simulink model "simuDosValvula"  (R2018a)
settings: Solver=VariableStepAuto  StartTime=0.0  StopTime=2  RelTol=1e-3
libraries: simulink x2, pePwmGenerator x2, vrlib x1
settings Model: Creator=Ruben  LastModifiedBy=Ruben

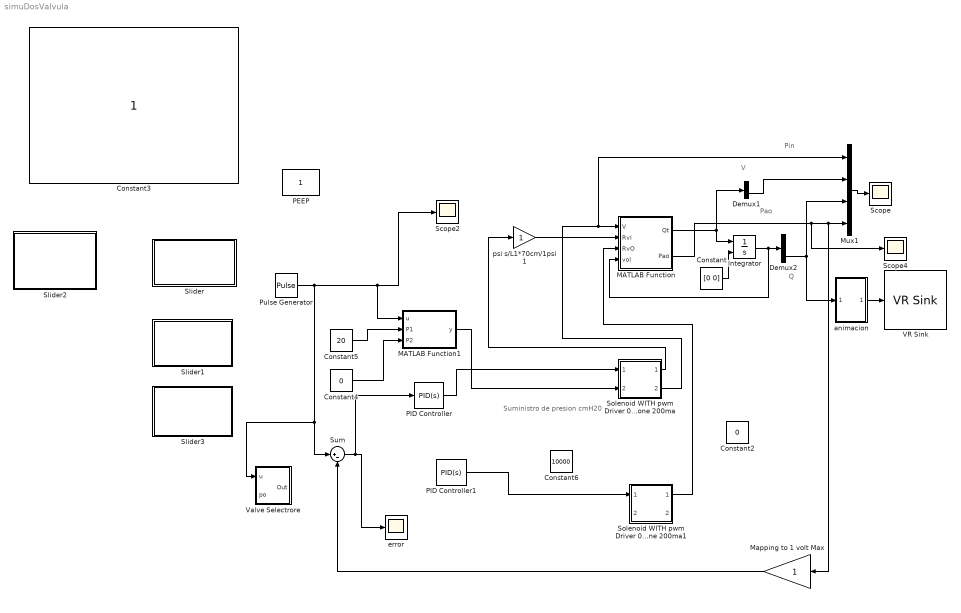
== system simuDosValvula ==
  note: Suministro de presion
      | cmH20
  note: Q
  note: Pin
  note: V
  note: Pao
  Constant : Constant  Value="[0    0]"
  Constant2 : Constant  Value=0
  Constant3 : Constant
      mask Display: image('C:\Users\Ruben\Downloads\Equivalente.png');
  Constant4 : Constant  Value=0
  Constant5 : Constant  Value=20
  Constant6 : Constant  Value=10000
  Demux1 : Demux  Outputs=2
  Demux2 : Demux  Outputs=2
  Integrator : Integrator  InitialConditionSource=external
  MATLAB Function : MATLAB Function  TreatAsAtomicUnit=on
  MATLAB Function1 : MATLAB Function  TreatAsAtomicUnit=on
  Mapping to 1 volt Max : Gain
  Mux1 : Mux
  PEEP : Constant
  PID Controller : simulink/Continuous/PID Controller  Controller=PID  TimeDomain=Continuous-time  SampleTime=-1  IntegratorMethod=Forward Euler  FilterMethod=Forward Euler  Form=Parallel  UseFilter=on  ControllerParametersSource=internal  P=.05  I=0  D=0  N=100  InitialConditionSource=internal  InitialConditionForIntegrator=0  InitialConditionForFilter=0  ExternalReset=none  LimitOutput=on  UpperSaturationLimit=1  LowerSaturationLimit=0  LinearizeAsGain=on  AntiWindupMode=none  Kb=1  TrackingMode=off  Kt=1  PParamMin=[]  PParamMax=[]  IParamMin=[]  IParamMax=[]  DParamMin=[]  DParamMax=[]  NParamMin=[]  NParamMax=[]  KbParamMin=[]  KbParamMax=[]  KtParamMin=[]  KtParamMax=[]  POutMin=[]  POutMax=[]  IOutMin=[]  IOutMax=[]  DOutMin=[]  DOutMax=[]  NOutMin=[]  NOutMax=[]  KbOutMin=[]  KbOutMax=[]  KtOutMin=[]  KtOutMax=[]  IntegratorOutMin=[]  IntegratorOutMax=[]  FilterOutMin=[]  FilterOutMax=[]  SumOutMin=[]  SumOutMax=[]  SumI1OutMin=[]  SumI1OutMax=[]  SumI2OutMin=[]  SumI2OutMax=[]  SumI3OutMin=[]  SumI3OutMax=[]  SumDOutMin=[]  SumDOutMax=[]  SaturationOutMin=[]  SaturationOutMax=[]  IntegratorContinuousStateAttributes=''  IntegratorStateMustResolveToSignalObject=off  IntegratorRTWStateStorageClass=Auto  FilterContinuousStateAttributes=''  FilterStateMustResolveToSignalObject=off  FilterRTWStateStorageClass=Auto  DifferentiatorICPrevScaledInput=0  DifferentiatorOutMin=[]  DifferentiatorOutMax=[]  FilterDiffOutCoefMin=[]  FilterDiffOutCoefMax=[]  SumDenOutMin=[]  SumDenOutMax=[]  SumNumOutMin=[]  SumNumOutMax=[]  ReciprocalOutMin=[]  ReciprocalOutMax=[]  DivideOutMin=[]  DivideOutMax=[]  TunerSelectOption=Transfer Function Based (PID Tuner App)
  PID Controller1 : simulink/Continuous/PID Controller  Controller=PID  TimeDomain=Continuous-time  SampleTime=-1  IntegratorMethod=Forward Euler  FilterMethod=Forward Euler  Form=Parallel  UseFilter=on  ControllerParametersSource=internal  P=1  I=0  D=0  N=100  InitialConditionSource=internal  InitialConditionForIntegrator=0  InitialConditionForFilter=0  ExternalReset=none  LimitOutput=on  UpperSaturationLimit=1  LowerSaturationLimit=0  LinearizeAsGain=on  AntiWindupMode=none  Kb=1  TrackingMode=off  Kt=1  PParamMin=[]  PParamMax=[]  IParamMin=[]  IParamMax=[]  DParamMin=[]  DParamMax=[]  NParamMin=[]  NParamMax=[]  KbParamMin=[]  KbParamMax=[]  KtParamMin=[]  KtParamMax=[]  POutMin=[]  POutMax=[]  IOutMin=[]  IOutMax=[]  DOutMin=[]  DOutMax=[]  NOutMin=[]  NOutMax=[]  KbOutMin=[]  KbOutMax=[]  KtOutMin=[]  KtOutMax=[]  IntegratorOutMin=[]  IntegratorOutMax=[]  FilterOutMin=[]  FilterOutMax=[]  SumOutMin=[]  SumOutMax=[]  SumI1OutMin=[]  SumI1OutMax=[]  SumI2OutMin=[]  SumI2OutMax=[]  SumI3OutMin=[]  SumI3OutMax=[]  SumDOutMin=[]  SumDOutMax=[]  SaturationOutMin=[]  SaturationOutMax=[]  IntegratorContinuousStateAttributes=''  IntegratorStateMustResolveToSignalObject=off  IntegratorRTWStateStorageClass=Auto  FilterContinuousStateAttributes=''  FilterStateMustResolveToSignalObject=off  FilterRTWStateStorageClass=Auto  DifferentiatorICPrevScaledInput=0  DifferentiatorOutMin=[]  DifferentiatorOutMax=[]  FilterDiffOutCoefMin=[]  FilterDiffOutCoefMax=[]  SumDenOutMin=[]  SumDenOutMax=[]  SumNumOutMin=[]  SumNumOutMax=[]  ReciprocalOutMin=[]  ReciprocalOutMax=[]  DivideOutMin=[]  DivideOutMax=[]  TunerSelectOption=Transfer Function Based (PID Tuner App)
  Pulse Generator : DiscretePulseGenerator  PulseType=Time based  Amplitude=10  Period=4  PulseWidth=30
  Scope : Scope
  Scope2 : Scope
  Scope4 : Scope
  Slider : Subsystem  DialogController=hmiCreateDDGDialog  IsWebBlock=on  mask(MWDashboardBlock){webBlockId=5c75009d-8c8d-43fb-88f0-46defad8d923, webBlockType=slider, ShowInLibBrowser=on, ShowInitialText=on, HMISrcModelName=simuDosValvula}
      mask prompts: webBlockId "WebBlock Id"; webBlockType "WebBlock Type"; HMISrcModelName "Source Model"
      mask help: SimulinkHMI:dialogs:SliderDialogDesc
      mask Help: helpview([docroot '/mapfiles/simulink.map'], 'hmi_slider')
      mask Display:
      | if strcmp(get_param(bdroot(gcb),'BlockDiagramType'), 'library')
      |     image([(matlabroot) '/toolbox/simulink/hmi/icons/Slider.png']);
      | end
  Slider1 : Subsystem  DialogController=hmiCreateDDGDialog  IsWebBlock=on  mask(MWDashboardBlock){webBlockId=99f10f40-54f3-4e18-818e-e2eb05ba8e4b, webBlockType=slider, ShowInLibBrowser=on, ShowInitialText=on, HMISrcModelName=simuDosValvula}
      mask prompts: webBlockId "WebBlock Id"; webBlockType "WebBlock Type"; HMISrcModelName "Source Model"
      mask help: SimulinkHMI:dialogs:SliderDialogDesc
      mask Help: helpview([docroot '/mapfiles/simulink.map'], 'hmi_slider')
      mask Display:
      | if strcmp(get_param(bdroot(gcb),'BlockDiagramType'), 'library')
      |     image([(matlabroot) '/toolbox/simulink/hmi/icons/Slider.png']);
      | end
  Slider2 : Subsystem  DialogController=hmiCreateDDGDialog  IsWebBlock=on  mask(MWDashboardBlock){webBlockId=e22ecaa3-1780-4869-841e-5d5c93829daa, webBlockType=slider, ShowInLibBrowser=on, ShowInitialText=on, HMISrcModelName=simuDosValvula}
      mask prompts: webBlockId "WebBlock Id"; webBlockType "WebBlock Type"; HMISrcModelName "Source Model"
      mask help: SimulinkHMI:dialogs:SliderDialogDesc
      mask Help: helpview([docroot '/mapfiles/simulink.map'], 'hmi_slider')
      mask Display:
      | if strcmp(get_param(bdroot(gcb),'BlockDiagramType'), 'library')
      |     image([(matlabroot) '/toolbox/simulink/hmi/icons/Slider.png']);
      | end
  Slider3 : Subsystem  DialogController=hmiCreateDDGDialog  IsWebBlock=on  mask(MWDashboardBlock){webBlockId=ff860e86-57b2-4262-afc4-ebabe2220a1a, webBlockType=slider, ShowInLibBrowser=on, ShowInitialText=on, HMISrcModelName=simuDosValvula}
      mask prompts: webBlockId "WebBlock Id"; webBlockType "WebBlock Type"; HMISrcModelName "Source Model"
      mask help: SimulinkHMI:dialogs:SliderDialogDesc
      mask Help: helpview([docroot '/mapfiles/simulink.map'], 'hmi_slider')
      mask Display:
      | if strcmp(get_param(bdroot(gcb),'BlockDiagramType'), 'library')
      |     image([(matlabroot) '/toolbox/simulink/hmi/icons/Slider.png']);
      | end
  Solenoid WITH pwm Driver 0v  closed to 1v fully  open min Resi=0.366 at 600ma (1 volt) dead zone 200ma : Subsystem  TreatAsAtomicUnit=on
      mask Display: image('C:\Users\Ruben\Downloads\Proportional-Safety_Valve.jpg');
  Solenoid WITH pwm Driver 0v  closed to 1v fully  open min Resi=0.366 at 600ma (1 volt) dead zone 200ma1 : Subsystem  TreatAsAtomicUnit=on
      mask Display: image('C:\Users\Ruben\Downloads\Proportional-Safety_Valve.jpg');
  Sum : Sum  Inputs=|+-
  VR Sink : vrlib/VR Sink  InstantiateOnLoad=on  SampleTime=0.1  ViewEnable=on  RemoteChange=off  RemoteView=off  FieldsWritten=lungs.scale.3.1.1.double  WorldFileName=Lungs2.wrl  AutoView=off  VideoDimensions=[]  AllowVariableSize=off  mask(Virtual Reality Sink){}
      settings: SourceProductBaseCode=VR
      mask Display: image('C:\Users\Ruben\Downloads\animacion.png');
  Valve Selectrore : MATLAB Function  TreatAsAtomicUnit=on
  animacion : Subsystem  TreatAsAtomicUnit=on
  error : Scope
  psi s/L1*70cm/1psi 1 : Gain
  wires:
  MATLAB Function/1(Qt) -> Integrator/1, Demux1/1
  Integrator/1 -> Demux2/1, MATLAB Function/4(vol)
  Constant/1 -> Integrator/2
  Solenoid WITH pwm Driver 0v  closed to 1v fully  open min Resi=0.366 at 600ma (1 volt) dead zone 200ma/1(Req(PSI.min/L)ma) -> psi s/L1*70cm/1psi 1/1
  psi s/L1*70cm/1psi 1/1 -> MATLAB Function/2(RvI)
  MATLAB Function1/1(y) -> Solenoid WITH pwm Driver 0v  closed to 1v fully  open min Resi=0.366 at 600ma (1 volt) dead zone 200ma/2(Pesion)
  Demux2/2 -> animacion/1(In1), Mux1/3
  Mux1/1 -> Scope/1
  Demux1/2 -> Mux1/2
  animacion/1(Out1) -> VR Sink/1
  Solenoid WITH pwm Driver 0v  closed to 1v fully  open min Resi=0.366 at 600ma (1 volt) dead zone 200ma/2(Presion) -> Mux1/1, MATLAB Function/1(V)
  Pulse Generator/1 -> Valve Selectrore/1(u), Sum/1, MATLAB Function1/1(u), Scope2/1
  MATLAB Function/2(Pao) -> Scope4/1, Mapping to 1 volt Max/1, Mux1/4
  Constant4/1 -> MATLAB Function1/3(P2)
  Constant5/1 -> MATLAB Function1/2(P1)
  Mapping to 1 volt Max/1 -> Sum/2
  Sum/1 -> PID Controller/1, error/1
  Solenoid WITH pwm Driver 0v  closed to 1v fully  open min Resi=0.366 at 600ma (1 volt) dead zone 200ma1/1(Req(PSI.min/L)ma) -> MATLAB Function/3(RvO)
  PID Controller/1 -> Solenoid WITH pwm Driver 0v  closed to 1v fully  open min Resi=0.366 at 600ma (1 volt) dead zone 200ma/1("Volts ")
  PID Controller1/1 -> Solenoid WITH pwm Driver 0v  closed to 1v fully  open min Resi=0.366 at 600ma (1 volt) dead zone 200ma1/1("Volts ")

== system simuDosValvula/Slider ==

== system simuDosValvula/Slider1 ==

== system simuDosValvula/Slider2 ==

== system simuDosValvula/Slider3 ==

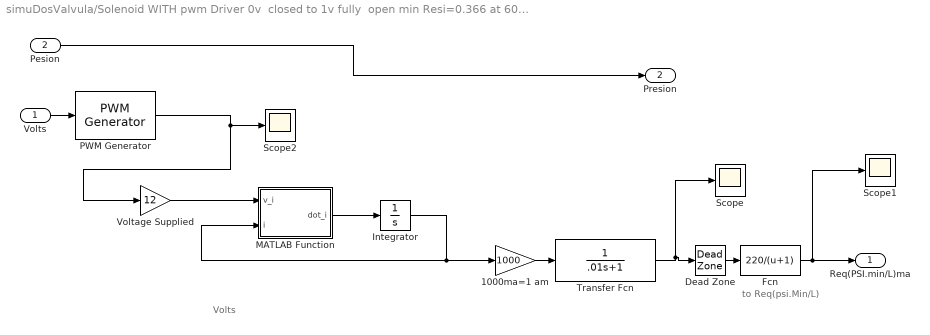
== system simuDosValvula/Solenoid WITH pwm Driver 0v  closed to 1v fully  open min Resi=0.366 at 600ma (1 volt) dead zone 200ma ==
  note: to Req(psi.Min/L)
  note: Volts
  "Volts " : Inport
  Pesion : Inport  Port=2
  1000ma=1 am : Gain  Gain=1000
  Dead Zone : DeadZone  LowerValue=0  UpperValue=0  SaturateOnIntegerOverflow=on
  Fcn : Fcn  Expr=220/(u+1)
  Integrator : Integrator
  MATLAB Function : MATLAB Function  TreatAsAtomicUnit=on
  PWM Generator : pePwmGenerator/PWM Generator  CarrCount=Up  Tper=0.001  Ts=5e-5
  Scope : Scope
  Scope1 : Scope
  Scope2 : Scope
  Transfer Fcn : TransferFcn  Denominator=[.01 1]
  Voltage Supplied : Gain  Gain=12
  Req(PSI.min/L)ma : Outport
  Presion : Outport  Port=2
  wires:
  Integrator/1 -> 1000ma=1 am/1, MATLAB Function/2(i)
  MATLAB Function/1(dot_i) -> Integrator/1
  1000ma=1 am/1 -> Transfer Fcn/1
  Fcn/1 -> Scope1/1, Req(PSI.min/L)ma/1
  Dead Zone/1 -> Fcn/1
  Transfer Fcn/1 -> Dead Zone/1, Scope/1
  PWM Generator/1 -> Voltage Supplied/1, Scope2/1
  "Volts "/1 -> PWM Generator/1
  Voltage Supplied/1 -> MATLAB Function/1(v_i)
  Pesion/1 -> Presion/1

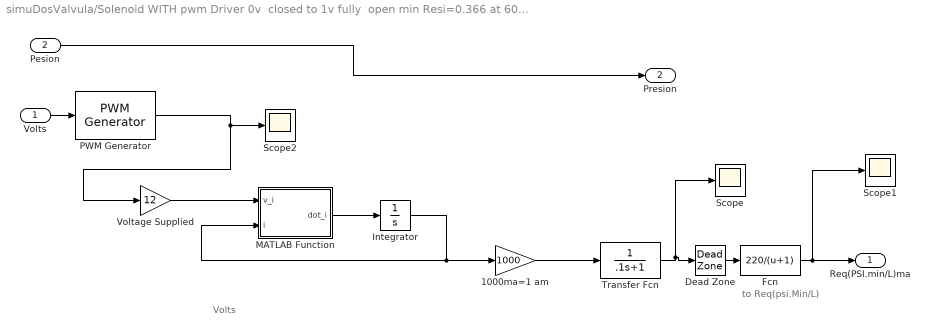
== system simuDosValvula/Solenoid WITH pwm Driver 0v  closed to 1v fully  open min Resi=0.366 at 600ma (1 volt) dead zone 200ma1 ==
  note: to Req(psi.Min/L)
  note: Volts
  "Volts " : Inport
  Pesion : Inport  Port=2
  1000ma=1 am : Gain  Gain=1000
  Dead Zone : DeadZone  LowerValue=0  UpperValue=200  SaturateOnIntegerOverflow=on
  Fcn : Fcn  Expr=220/(u+1)
  Integrator : Integrator
  MATLAB Function : MATLAB Function  TreatAsAtomicUnit=on
  PWM Generator : pePwmGenerator/PWM Generator  CarrCount=Up  Tper=0.1  Ts=5e-5
  Scope : Scope
  Scope1 : Scope
  Scope2 : Scope
  Transfer Fcn : TransferFcn  Denominator=[.1 1]
  Voltage Supplied : Gain  Gain=12
  Req(PSI.min/L)ma : Outport
  Presion : Outport  Port=2
  wires:
  Integrator/1 -> 1000ma=1 am/1, MATLAB Function/2(i)
  MATLAB Function/1(dot_i) -> Integrator/1
  1000ma=1 am/1 -> Transfer Fcn/1
  Fcn/1 -> Scope1/1, Req(PSI.min/L)ma/1
  Dead Zone/1 -> Fcn/1
  Transfer Fcn/1 -> Dead Zone/1, Scope/1
  PWM Generator/1 -> Voltage Supplied/1, Scope2/1
  "Volts "/1 -> PWM Generator/1
  Voltage Supplied/1 -> MATLAB Function/1(v_i)
  Pesion/1 -> Presion/1

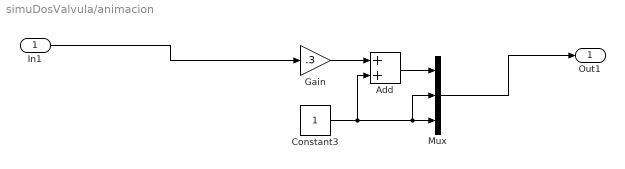
== system simuDosValvula/animacion ==
  In1 : Inport
  Add : Sum
  Constant3 : Constant
  Gain : Gain  Gain=.3
  Mux : Mux  Inputs=3
  Out1 : Outport
  wires:
  Constant3/1 -> Add/2, Mux/2, Mux/3
  In1/1 -> Gain/1
  Add/1 -> Mux/1
  Gain/1 -> Add/1
  Mux/1 -> Out1/1

== matlab function simuDosValvula/Solenoid WITH pwm Driver 0v  closed to 1v fully  open min Resi=0.366 at 600ma (1 volt) dead zone 200ma/MATLAB Function ==
  data: v_i input; dot_i output; i input
function dot_i = fcn(v_i,i)
R=15; % R igual a 2 ohm
%L=.063 ;% L aprox 63mh
%L=.063;
L=.006;

dot_i = (1/L)*(v_i-R*i);

== matlab function simuDosValvula/MATLAB Function ==
  data: V input; RvI input; RvO input; Qt output; vol input; Pao output
function [Qt,Pao]  = fcn(V,RvI,RvO,vol)
intI2=vol(1);
intI3=vol(2);
RVV=(RvI*RvO)/(RvI+RvO);
Rc=1;Rp=1; %R1=RC,R2=Rp
%Cs=.005;Cl=0.2; Cw=0.2;%C1=Cs; C2=Cl*CW
Cs=.005;Cl=0.2; Cw=0.2;%C1=Cs; C2=Cl*CW
%Q=I3,Qa=I2



%C2=Cl+Cw
Q=(1/(Rc+RVV))*(V-(1/Cs)*(-intI2+intI3));
Qa=(1/Rp)*(V-Q*(Rc+RVV)-(1/(Cl+Cw))*intI2);

Pao=V-Q*RVV;
Qt = [ Qa  Q];

== matlab function simuDosValvula/Solenoid WITH pwm Driver 0v  closed to 1v fully  open min Resi=0.366 at 600ma (1 volt) dead zone 200ma1/MATLAB Function ==
  data: v_i input; dot_i output; i input
function dot_i = fcn(v_i,i)
R=15; % R igual a 2 ohm
%L=.063 ;% L aprox 63mh
L=.063;
dot_i = (1/L)*(v_i-R*i);

== matlab function simuDosValvula/MATLAB Function1 ==
  data: u input; y output; P1 input; P2 input
function y = fcn(u,P1,P2)
if u > 5 
   y = P1;
else
    y=  P2;
    
    
end

== matlab function simuDosValvula/Valve Selectrore ==
  data: u input; Out output; po input
function Out = fcn(u,po)
if     u > 5
     
     Out=0;
else      

Out=-(u-po);
end
